simulink model "imuposition"  (Simulink 7.5)
settings: Solver=ode3  StartTime=0.0  StopTime=inf  FixedStep=.05  RelTol=1e-3
undefined symbols (not defined in the file or in its folder): CR, serial
libraries: instrumentlib x2, realtime_pacer_lib x1
settings Model: Creator=TCA  LastModifiedBy=meuser
settings OptimizationCC: InitFltsAndDblsToZero=on
settings DebuggingCC: StrictBusMsg=Warning

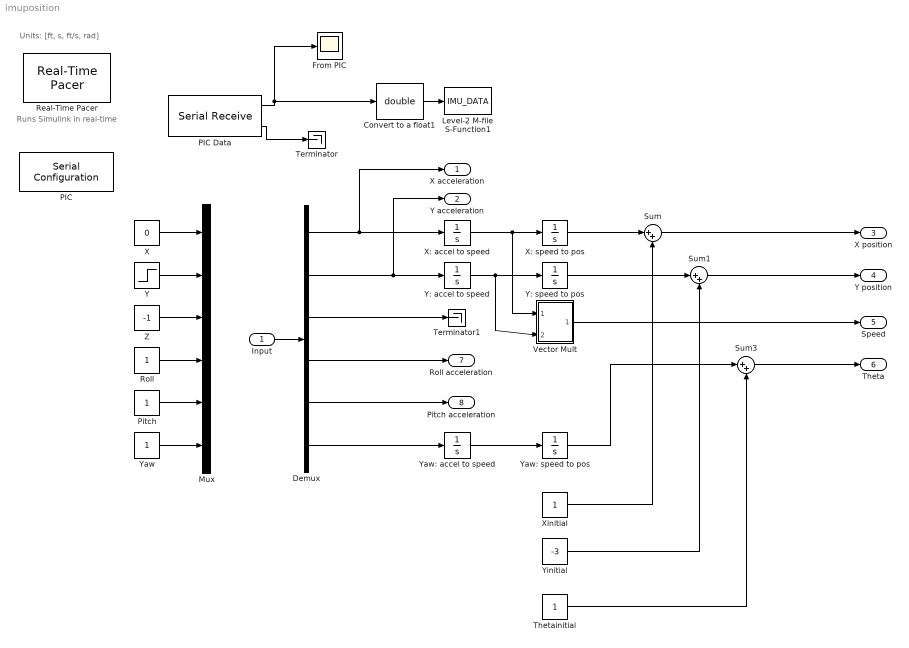
== system imuposition ==
  note: Runs Simulink
      |  in real-time
  note: Units: [ft, s, ft/s, rad]
  Input : Inport  OutDataType=fixdt(1, 16)  OutScaling=2^0
  Convert to a float1 : DataTypeConversion  OutDataTypeMode=double  OutDataTypeStr=double  SaturateOnIntegerOverflow=on  RndMeth=Zero
  Demux : Demux  Outputs=6
  From PIC : Scope
      settings: TimeRange=10  YMin=0  YMax=250
  Level-2 M-file S-Function1 : M-S-Function  FunctionName=IMU_DATA  Parameters=1
  Mux : Mux  Inputs=6
  PIC : instrumentlib/Serial Configuration  Priority=-200000  DialogController=instrumentcreatedialog  DialogControllerArgs=DataTag0  ComPortMenu=COM6  ComPort=COM6  ObjConstructor=serial('COM6');  BaudRate=9600  DataBits=8  Parity=none  StopBits=1  FlowControl=none  Timeout=10  ByteOrder=LittleEndian
  PIC Data : instrumentlib/Serial Receive  DialogController=instrumentcreatedialog  DialogControllerArgs=DataTag1  ComPortMenu=COM6  ComPort=COM6  ObjConstructor=serial('COM6');  Terminator=CR ('\r')  DataSize="[1  12]"  DataType=uint8  EnableBlockingMode=off  ActionDataUnavailable=Output last received value  CustomValue=0  SampleTime=.05
  Pitch : Constant  OutDataType=fixdt(1, 16)  OutScaling=2^0
  Real-Time Pacer : realtime_pacer_lib/Real-Time Pacer  simTimePerRealTime=1
  Roll : Constant  OutDataType=fixdt(1, 16)  OutScaling=2^0
  Sum : Sum  Inputs=|++  OutDataType=fixdt(1, 16)  OutScaling=2^0
  Sum1 : Sum  Inputs=|++  OutDataType=fixdt(1, 16)  OutScaling=2^0
  Sum3 : Sum  Inputs=|++  OutDataType=fixdt(1, 16)  OutScaling=2^0
  Terminator : Terminator
  Terminator1 : Terminator
  Thetainitial : Constant  OutDataType=fixdt(1, 16)  OutScaling=2^0
  Vector Mult : Subsystem
  X : Constant  Value=0  OutDataType=fixdt(1, 16)  OutScaling=2^0
  X: accel to speed : Integrator
  X: speed to pos : Integrator
  Xinitial : Constant  OutDataType=fixdt(1, 16)  OutScaling=2^0
  Y : Step  Time=3  After=2  SampleTime=0
  Y: accel to speed : Integrator
  Y: speed to pos : Integrator
  Yaw : Constant  OutDataType=fixdt(1, 16)  OutScaling=2^0
  Yaw: accel to speed : Integrator
  Yaw: speed to pos : Integrator
  Yinitial : Constant  Value=-3  OutDataType=fixdt(1, 16)  OutScaling=2^0
  Z : Constant  Value=-1  OutDataType=fixdt(1, 16)  OutScaling=2^0
  X acceleration : Outport  OutDataType=fixdt(1, 16)  OutScaling=2^0
  Y acceleration : Outport  Port=2  OutDataType=fixdt(1, 16)  OutScaling=2^0
  X position : Outport  Port=3  OutDataType=fixdt(1, 16)  OutScaling=2^0
  Y position : Outport  Port=4  OutDataType=fixdt(1, 16)  OutScaling=2^0
  Speed : Outport  Port=5  OutDataType=fixdt(1, 16)  OutScaling=2^0
  Theta : Outport  Port=6  OutDataType=fixdt(1, 16)  OutScaling=2^0
  Roll acceleration : Outport  Port=7  OutDataType=fixdt(1, 16)  OutScaling=2^0
  Pitch acceleration : Outport  Port=8  OutDataType=fixdt(1, 16)  OutScaling=2^0
  wires:
  Convert to a float1/1 -> Level-2 M-file S-Function1/1
  PIC Data/1 -> From PIC/1, Convert to a float1/1
  PIC Data/2 -> Terminator/1
  X/1 -> Mux/1
  Y/1 -> Mux/2
  Z/1 -> Mux/3
  Roll/1 -> Mux/4
  Pitch/1 -> Mux/5
  Yaw/1 -> Mux/6
  Vector Mult/1(Speed) -> Speed/1
  Sum3/1 -> Theta/1
  Yaw: speed to pos/1 -> Sum3/1
  Thetainitial/1 -> Sum3/2
  Yinitial/1 -> Sum1/2
  Xinitial/1 -> Sum/2
  Demux/6 -> Yaw: accel to speed/1
  Demux/5 -> Pitch acceleration/1
  Demux/4 -> Roll acceleration/1
  Yaw: accel to speed/1 -> Yaw: speed to pos/1
  Sum1/1 -> Y position/1
  Sum/1 -> X position/1
  X: speed to pos/1 -> Sum/1
  Y: speed to pos/1 -> Sum1/1
  Y: accel to speed/1 -> Y: speed to pos/1, Vector Mult/2(Y-vel)
  X: accel to speed/1 -> X: speed to pos/1, Vector Mult/1(X-vel)
  Demux/3 -> Terminator1/1
  Demux/2 -> Y: accel to speed/1, Y acceleration/1
  Demux/1 -> X: accel to speed/1, X acceleration/1
  Input/1 -> Demux/1

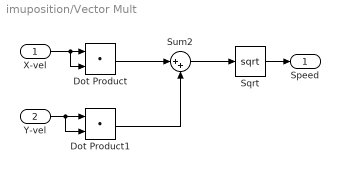
== system imuposition/Vector Mult ==
  X-vel : Inport
  Y-vel : Inport  Port=2
  Dot Product : DotProduct  OutDataType=fixdt(1, 16)  OutScaling=2^-10  InputSameDT=on  OutDataTypeStr=Inherit: Inherit via internal rule
  Dot Product1 : DotProduct  OutDataType=fixdt(1, 16)  OutScaling=2^-10  InputSameDT=on  OutDataTypeStr=Inherit: Inherit via internal rule
  Sqrt : Sqrt  SaturateOnIntegerOverflow=on
  Sum2 : Sum  Inputs=|++  OutDataType=fixdt(1, 16)  OutScaling=2^0
  Speed : Outport
  wires:
  Dot Product1/1 -> Sum2/2
  Dot Product/1 -> Sum2/1
  Sum2/1 -> Sqrt/1
  X-vel/1 -> Dot Product/1, Dot Product/2
  Sqrt/1 -> Speed/1
  Y-vel/1 -> Dot Product1/1, Dot Product1/2
